simulink model "Torque_Vectoring"  (R2024a)
settings: Solver=FixedStepAuto  StartTime=0.0  StopTime=10.0  FixedStep=0.01  RelTol=1e-3
model workspace (MAT data in the model file):
  diff_table_F = [0 0.0005 0.0005 0.0006 0.0006 0.0007 0.0008 0.0008 0.0009 0.0009 0.001 0.0011 0.0011 0.0012 0.0013 0.0014 0.0014 0.0015 0.0016 0.0017 0.0018 0.0018 0.0019 0.002 0.0021 0.0022 0.0023 0.0024 0.0025 0.0026 0.0027 0.0027 0.0028 0.0029 0.0031 0.0032 0.0033 0.0034 0.0035 0.0036 0.0037 0.0038 0.0039 0.004 0.0042 0.0043 0.0044 0.0045 0.0046 0.0048 0.0049 0.005 0.0051 0.0053 0.0054 0.0055 0.0057 0.0058 0.0059 0.0061 0.0062 0.0064 0.0065 0.0067 0.0068 0.007 0.0071 0.0073 0.0074 0.0076 0.0077 0.0079 0.008 0.0082 0.0084 0.0085 0.0087 0.0089 0.009 0.0092 0.0094 0.0095]
  diff_table_R = [0 0.0023 0.00253 0.00276 0.00299 0.00322 0.00345 0.00368 0.00391 0.00414 0.00437 0.0046 0.00483 0.00506 0.00529 0.00552 0.00575 0.00598 0.00621 0.00644 0.00667 0.0069 0.00713 0.00736 0.00759 0.00782 0.00805 0.00828 0.00851 0.00874 0.00897 0.0092 0.00943 0.00966 0.00989 0.01012 0.01035 0.01058 0.01081 0.01104 0.01127 0.0115 0.01173 0.01196 0.01219 0.01242 0.01265 0.01288 0.01311 0.01334 0.01357 0.0138 0.01403 0.01426 0.01449 0.01472 0.01495 0.01518 0.01541 0.01564 0.01587 0.0161 0.01633 0.01656 0.01679 0.01702 0.01725 0.01748 0.01771 0.01794 0.01817 0.0184 0.01863 0.01886 0.01909 0.01932 0.01955 0.01978 0.02001 0.02024 0.02047 0.0207]
  diff_table_ext_F = [0 0.0005 0.0005 0.0006 0.0006 0.0007 0.0008 0.0008 0.0009 0.0009 0.001 0.0011 0.0011 0.0012 0.0013 0.0014 0.0014 0.0015 0.0016 0.0017 0.0018 0.0018 0.0019 0.002 0.0021 0.0022 0.0023 0.0024 0.0025 0.0026 0.0027 0.0027 0.0028 0.0029 0.0031 0.0032 0.0033 0.0034 0.0035 0.0036 0.0037 0.0038 0.0039 0.004 0.0042 0.0043 0.0044 0.0045 0.0046 0.0048 0.0049 0.005 0.0051 0.0053 0.0054 0.0055 0.0057 0.0058 0.0059 0.0061 0.0062 0.0064 0.0065 0.0067 0.0068 0.007 0.0071 0.0073 0.0074 0.0076 0.0077 0.0079 0.008 0.0082 0.0084 0.0085 0.0087 0.0089 0.009 0.0092 0.0094 0.0095 0.0097 0.0099 0.01 0.0102 0.0104 0.0105 0.0107 0.0109 0.011 0.0112 0.0114 0.0115 0.0117 0.0119 0.012 0.0122 0.0124 0.0125 0.0127]
  diff_table_ext_R = [0 0.0023 0.00253 0.00276 0.00299 0.00322 0.00345 0.00368 0.00391 0.00414 0.00437 0.0046 0.00483 0.00506 0.00529 0.00552 0.00575 0.00598 0.00621 0.00644 0.00667 0.0069 0.00713 0.00736 0.00759 0.00782 0.00805 0.00828 0.00851 0.00874 0.00897 0.0092 0.00943 0.00966 0.00989 0.01012 0.01035 0.01058 0.01081 0.01104 0.01127 0.0115 0.01173 0.01196 0.01219 0.01242 0.01265 0.01288 0.01311 0.01334 0.01357 0.0138 0.01403 0.01426 0.01449 0.01472 0.01495 0.01518 0.01541 0.01564 0.01587 0.0161 0.01633 0.01656 0.01679 0.01702 0.01725 0.01748 0.01771 0.01794 0.01817 0.0184 0.01863 0.01886 0.01909 0.01932 0.01955 0.01978 0.02001 0.02024 0.02047 0.0207 0.02093 0.02116 0.02139 0.02162 0.02185 0.02208 0.02231 0.02254 0.02277 0.023 0.02323 0.02346 0.02369 0.02392 0.02415 0.02438 0.02461 0.02484 0.02507]
undefined symbols (not defined in the file): accX, accY, amk_actual_speed, base_torques, dash_se, diff_gain_n, diff_gain_outer, fl, fr, gyrZ, max_torque_front, max_torque_rear, min_torque_front, min_torque_rear, newsignal1, rl, rr, te_main_APPS, te_main_BPSe, torque_front_n, torque_front_p, torque_rear_n, torque_rear_p, yrc_diff_gain, yrc_grip, yrc_ki, yrc_kp_acc, yrc_kp_regen, yrc_ku, yrc_lambda1, yrc_lambda2, yrc_lambda3, yrc_max_power, yrc_steer_factor
libraries: simulink_extras x1, slpidlib x1
settings Model: Creator=andre  LastModifiedBy=pedro
settings OptimizationCC: ZeroExternalMemoryAtStartup=off  ZeroInternalMemoryAtStartup=off
settings RTWCC: Toolchain=Colcon Tools  TargetLang=C++
settings GRTTargetCC: TargetLangStandard=C++11 (ISO)  CodeInterfacePackaging=C++ class  MultiInstanceErrorCode=Warning

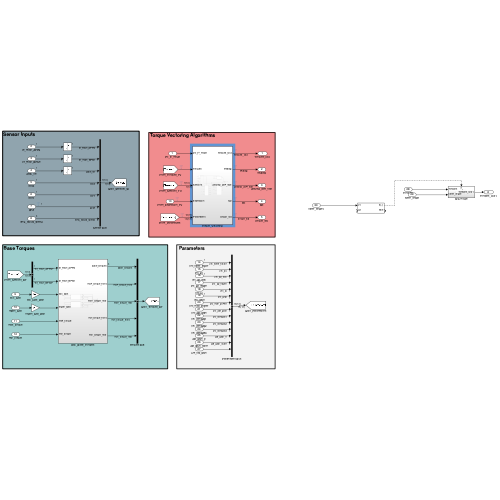
[thumbnail: Simulink's stored preview of the top-level diagram]
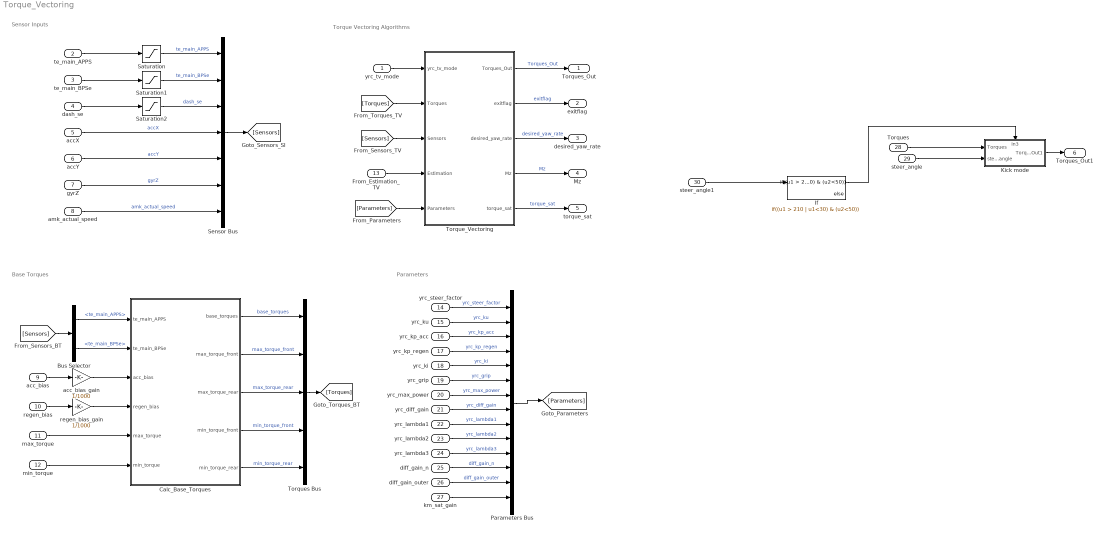
== system Torque_Vectoring ==
  note: Parameters
  note: Base Torques
  note: Torque Vectoring Algorithms
  note: Sensor Inputs
  yrc_tv_mode : Inport
  te_main_APPS : Inport  Port=2  PortDimensions=1
  te_main_BPSe : Inport  Port=3  PortDimensions=1
  dash_se : Inport  Port=4  PortDimensions=1
  accX : Inport  Port=5  PortDimensions=1
  accY : Inport  Port=6  PortDimensions=1
  gyrZ : Inport  Port=7  PortDimensions=1
  amk_actual_speed : Inport  Port=8  PortDimensions=4
  acc_bias : Inport  Port=9
  regen_bias : Inport  Port=10
  max_torque : Inport  Port=11
  min_torque : Inport  Port=12
  From_Estimation_TV : Inport  Port=13
  yrc_steer_factor : Inport  Port=14  PortDimensions=1
  yrc_ku : Inport  Port=15  PortDimensions=1
  yrc_kp_acc : Inport  Port=16  PortDimensions=1
  yrc_kp_regen : Inport  Port=17  PortDimensions=1
  yrc_ki : Inport  Port=18  PortDimensions=1
  yrc_grip : Inport  Port=19  PortDimensions=1
  yrc_max_power : Inport  Port=20  PortDimensions=1
  yrc_diff_gain : Inport  Port=21  PortDimensions=1
  yrc_lambda1 : Inport  Port=22  PortDimensions=1
  yrc_lambda2 : Inport  Port=23  PortDimensions=1
  yrc_lambda3 : Inport  Port=24  PortDimensions=1
  diff_gain_n : Inport  Port=25  PortDimensions=1
  diff_gain_outer : Inport  Port=26  PortDimensions=1
  km_sat_gain : Inport  Port=27
  Torques : Inport  Port=28
  steer_angle : Inport  Port=29
  steer_angle1 : Inport  Port=30
  Bus Selector : BusSelector  OutputSignals=te_main_APPS,te_main_BPSe
  Calc_Base_Torques : Subsystem
  If : If  NumInputs=2  IfExpression=(u1 > 210 | u1<30) & (u2<50)
  Kick mode : Subsystem
      settings: PortSchema="{\"entries\":[{\"content\":{\"sides\":[{\"content\":{\"connectorIds\":[\"In1\",\"In2\"]},\"type\":\"ConnectorPlacement.EquallySpacedRectSide\",\"uuid\":\"e9897e70-c7c7-4947-a7d8-b7fe2c92736f\"},{\"content\":{\"connectorIds\":[\"Out1\"],\"side\":\"RIGHT\"},\"type\":\"ConnectorPlacement.EquallySpacedRectSide\",\"uuid\":\"5825815b-03a9-422c-b961-b03bf00c9827\"},{\"content\":{\"connectorIds\":[\"In3\"],\"side\":\"TOP\"},\"type\":\"ConnectorPlacement.EquallySpacedRectSide\",\"uuid\":\"e2faf393-33b7-422a-8f4d-99abbde724a7\"}]},\"type\":\"ConnectorPlacement.EquallySpacedConnector\",\"uuid\":\"5fc9237a-4862-4d27-81be-376c484d3dd1\"}],\"packageUris\":[\"http://schema.mathworks.com/mf0/Connector/R2020b\"],\"version\":\"1.0\"}"
  Parameters Bus : BusCreator  Inputs=yrc_steer_factor,yrc_ku,yrc_kp_acc,yrc_kp_regen,yrc_ki,yrc_grip,yrc_max_power,yrc_diff_gain,yrc_lambda1,yrc_lambda2,yrc_lambda3,diff_gain_n,diff_gain_outer,newsignal1
  Saturation : Saturate  UpperLimit=100  LowerLimit=0
  Saturation1 : Saturate  UpperLimit=100  LowerLimit=0
  Saturation2 : Saturate  UpperLimit=127  LowerLimit=-127
  Sensor Bus : BusCreator  Inputs=te_main_APPS,te_main_BPSe,dash_se,accX,accY,gyrZ,amk_actual_speed
  Torque_Vectoring : Subsystem
  Torques Bus : BusCreator  Inputs=base_torques,max_torque_front,max_torque_rear,min_torque_front,min_torque_rear
  acc_bias_gain : Gain  Gain=1/1000
  regen_bias_gain : Gain  Gain=1/1000
  Torques_Out : Outport
  exitflag : Outport  Port=2
  desired_yaw_rate : Outport  Port=3
  Mz : Outport  Port=4
  torque_sat : Outport  Port=5
  Torques_Out1 : Outport  Port=6
  wires:
  amk_actual_speed/1 -> Sensor Bus/7  "amk_actual_speed"
  Sensor Bus/1 -> [Sensors]
  yrc_grip/1 -> Parameters Bus/6  "yrc_grip"
  [Parameters] -> Torque_Vectoring/5(Parameters)
  [Torques] -> Torque_Vectoring/2(Torques)
  Torque_Vectoring/3(desired_yaw_rate) -> desired_yaw_rate/1  "desired_yaw_rate"
  regen_bias_gain/1 -> Calc_Base_Torques/4(regen_bias)
  Calc_Base_Torques/5(min_torque_rear) -> Torques Bus/5  "min_torque_rear"
  Calc_Base_Torques/4(min_torque_front) -> Torques Bus/4  "min_torque_front"
  yrc_max_power/1 -> Parameters Bus/7  "yrc_max_power"
  Bus Selector/1 -> Calc_Base_Torques/1(te_main_APPS)  "<te_main_APPS>"
  accY/1 -> Sensor Bus/5  "accY"
  Torque_Vectoring/5(torque_sat) -> torque_sat/1  "torque_sat"
  [Sensors] -> Bus Selector/1
  yrc_kp_regen/1 -> Parameters Bus/4  "yrc_kp_regen"
  Calc_Base_Torques/1(base_torques) -> Torques Bus/1  "base_torques"
  yrc_tv_mode/1 -> Torque_Vectoring/1(yrc_tv_mode)
  [Sensors] -> Torque_Vectoring/3(Sensors)
  Torques Bus/1 -> [Torques]
  regen_bias/1 -> regen_bias_gain/1
  Saturation1/1 -> Sensor Bus/2  "te_main_BPSe"
  dash_se/1 -> Saturation2/1
  yrc_ki/1 -> Parameters Bus/5  "yrc_ki"
  yrc_steer_factor/1 -> Parameters Bus/1  "yrc_steer_factor"
  min_torque/1 -> Calc_Base_Torques/6(min_torque)
  acc_bias/1 -> acc_bias_gain/1
  acc_bias_gain/1 -> Calc_Base_Torques/3(acc_bias)
  Calc_Base_Torques/2(max_torque_front) -> Torques Bus/2  "max_torque_front"
  te_main_APPS/1 -> Saturation/1
  Calc_Base_Torques/3(max_torque_rear) -> Torques Bus/3  "max_torque_rear"
  From_Estimation_TV/1 -> Torque_Vectoring/4(Estimation)
  Saturation/1 -> Sensor Bus/1  "te_main_APPS"
  yrc_kp_acc/1 -> Parameters Bus/3  "yrc_kp_acc"
  gyrZ/1 -> Sensor Bus/6  "gyrZ"
  Parameters Bus/1 -> [Parameters]
  Saturation2/1 -> Sensor Bus/3  "dash_se"
  accX/1 -> Sensor Bus/4  "accX"
  Bus Selector/2 -> Calc_Base_Torques/2(te_main_BPSe)  "<te_main_BPSe>"
  max_torque/1 -> Calc_Base_Torques/5(max_torque)
  te_main_BPSe/1 -> Saturation1/1
  Torque_Vectoring/4(Mz) -> Mz/1  "Mz"
  Torque_Vectoring/2(exitflag) -> exitflag/1  "exitflag"
  yrc_diff_gain/1 -> Parameters Bus/8  "yrc_diff_gain"
  yrc_ku/1 -> Parameters Bus/2  "yrc_ku"
  yrc_lambda1/1 -> Parameters Bus/9  "yrc_lambda1"
  yrc_lambda2/1 -> Parameters Bus/10  "yrc_lambda2"
  yrc_lambda3/1 -> Parameters Bus/11  "yrc_lambda3"
  diff_gain_n/1 -> Parameters Bus/12  "diff_gain_n"
  diff_gain_outer/1 -> Parameters Bus/13  "diff_gain_outer"
  Torque_Vectoring/1(Torques_Out) -> Torques_Out/1  "Torques_Out"
  km_sat_gain/1 -> Parameters Bus/14
  steer_angle1/1 -> If/1
  Kick mode/1(Torques_Out1) -> Torques_Out1/1
  If/1 -> Kick mode/3(In3)
  steer_angle/1 -> Kick mode/2(steer_angle)
  Torques/1 -> Kick mode/1(Torques)

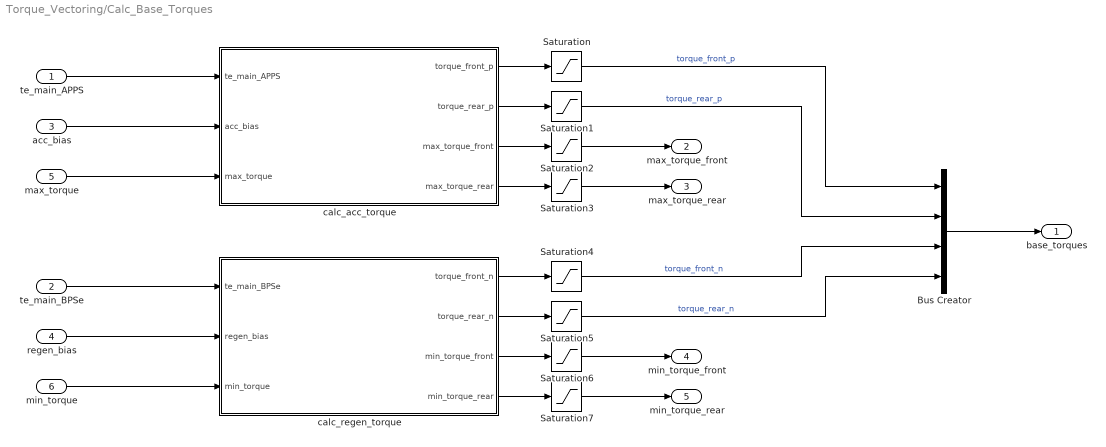
== system Torque_Vectoring/Calc_Base_Torques ==
  te_main_APPS : Inport
  te_main_BPSe : Inport  Port=2
  acc_bias : Inport  Port=3
  regen_bias : Inport  Port=4
  max_torque : Inport  Port=5
  min_torque : Inport  Port=6
  Bus Creator : BusCreator  Inputs=torque_front_p,torque_rear_p,torque_front_n,torque_rear_n
  Saturation{,1..3} (4 alike) : Saturate  UpperLimit=21000  LowerLimit=0
  Saturation{4..7} (4 alike) : Saturate  UpperLimit=0  LowerLimit=-21000
  calc_acc_torque : MATLAB Function  TreatAsAtomicUnit=on
  calc_regen_torque : MATLAB Function  TreatAsAtomicUnit=on
  base_torques : Outport  PortDimensions=4
  max_torque_front : Outport  Port=2
  max_torque_rear : Outport  Port=3
  min_torque_front : Outport  Port=4
  min_torque_rear : Outport  Port=5
  wires:
  te_main_APPS/1 -> calc_acc_torque/1(te_main_APPS)
  acc_bias/1 -> calc_acc_torque/2(acc_bias)
  max_torque/1 -> calc_acc_torque/3(max_torque)
  te_main_BPSe/1 -> calc_regen_torque/1(te_main_BPSe)
  regen_bias/1 -> calc_regen_torque/2(regen_bias)
  min_torque/1 -> calc_regen_torque/3(min_torque)
  calc_acc_torque/1(torque_front_p) -> Saturation/1
  calc_acc_torque/2(torque_rear_p) -> Saturation1/1
  calc_acc_torque/3(max_torque_front) -> Saturation2/1
  calc_acc_torque/4(max_torque_rear) -> Saturation3/1
  calc_regen_torque/1(torque_front_n) -> Saturation4/1
  calc_regen_torque/2(torque_rear_n) -> Saturation5/1
  calc_regen_torque/3(min_torque_front) -> Saturation6/1
  calc_regen_torque/4(min_torque_rear) -> Saturation7/1
  Saturation2/1 -> max_torque_front/1
  Saturation3/1 -> max_torque_rear/1
  Saturation6/1 -> min_torque_front/1
  Saturation7/1 -> min_torque_rear/1
  Bus Creator/1 -> base_torques/1
  Saturation/1 -> Bus Creator/1  "torque_front_p"
  Saturation1/1 -> Bus Creator/2  "torque_rear_p"
  Saturation4/1 -> Bus Creator/3  "torque_front_n"
  Saturation5/1 -> Bus Creator/4  "torque_rear_n"

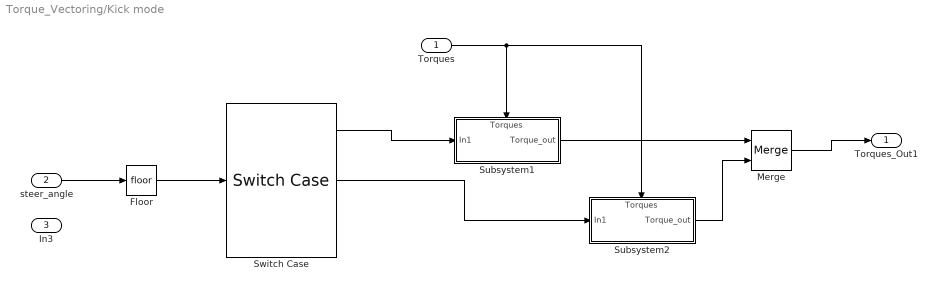
== system Torque_Vectoring/Kick mode ==
  Torques : Inport
  steer_angle : Inport  Port=2
  In3 : Inport  Port=3
  Floor : Rounding
  Merge : Merge
  Subsystem1 : Subsystem
      settings: PortSchema="{\"entries\":[{\"content\":{\"sides\":[{\"content\":{\"connectorIds\":[\"In1\"]},\"type\":\"ConnectorPlacement.EquallySpacedRectSide\",\"uuid\":\"08cef44f-9403-4a7e-80cd-188495bf4ffe\"},{\"content\":{\"connectorIds\":[\"Out1\"],\"side\":\"RIGHT\"},\"type\":\"ConnectorPlacement.EquallySpacedRectSide\",\"uuid\":\"56e69b5d-38a8-4864-8637-0441600913d6\"},{\"content\":{\"connectorIds\":[\"In2\"],\"side\":\"TOP\"},\"type\":\"ConnectorPlacement.EquallySpacedRectSide\",\"uuid\":\"983275be-1625-4fe8-b202-c3acafa806fd\"}]},\"type\":\"ConnectorPlacement.EquallySpacedConnector\",\"uuid\":\"3a10482c-ca03-43ee-b56a-b119a43dac9c\"}],\"packageUris\":[\"http://schema.mathworks.com/mf0/Connector/R2020b\"],\"version\":\"1.0\"}"
  Subsystem2 : Subsystem
      settings: PortSchema="{\"entries\":[{\"content\":{\"sides\":[{\"content\":{\"connectorIds\":[\"In1\"]},\"type\":\"ConnectorPlacement.EquallySpacedRectSide\",\"uuid\":\"08cef44f-9403-4a7e-80cd-188495bf4ffe\"},{\"content\":{\"connectorIds\":[\"Out1\"],\"side\":\"RIGHT\"},\"type\":\"ConnectorPlacement.EquallySpacedRectSide\",\"uuid\":\"56e69b5d-38a8-4864-8637-0441600913d6\"},{\"content\":{\"connectorIds\":[\"In2\"],\"side\":\"TOP\"},\"type\":\"ConnectorPlacement.EquallySpacedRectSide\",\"uuid\":\"983275be-1625-4fe8-b202-c3acafa806fd\"}]},\"type\":\"ConnectorPlacement.EquallySpacedConnector\",\"uuid\":\"3a10482c-ca03-43ee-b56a-b119a43dac9c\"}],\"packageUris\":[\"http://schema.mathworks.com/mf0/Connector/R2020b\"],\"version\":\"1.0\"}"
  Switch Case : SwitchCase  CaseConditions={[210:240],[0:30]}
  Torques_Out1 : Outport
  wires:
  Torques/1 -> Subsystem2/2(Torques), Subsystem1/2(Torques)
  steer_angle/1 -> Floor/1
  Floor/1 -> Switch Case/1
  Switch Case/1 -> Subsystem1/1(In1)
  Switch Case/2 -> Subsystem2/1(In1)
  Subsystem1/1(Torque_out) -> Merge/1
  Subsystem2/1(Torque_out) -> Merge/2
  Merge/1 -> Torques_Out1/1

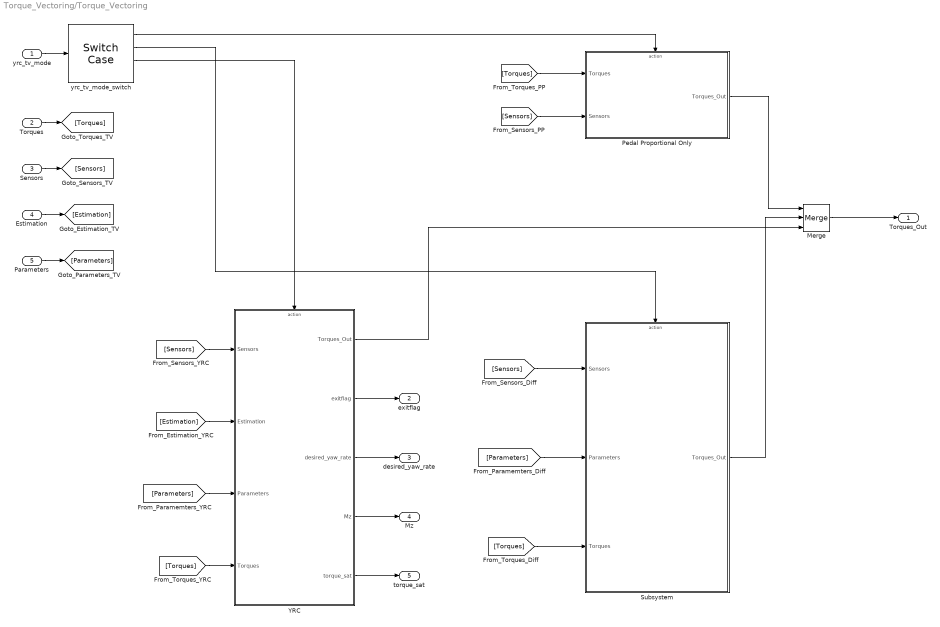
== system Torque_Vectoring/Torque_Vectoring ==
  yrc_tv_mode : Inport
  Torques : Inport  Port=2
  Sensors : Inport  Port=3
  Estimation : Inport  Port=4
  Parameters : Inport  Port=5
  Merge : Merge  Inputs=3
  Pedal Proportional Only : Subsystem
  Subsystem : Subsystem
  YRC : Subsystem
  yrc_tv_mode_switch : SwitchCase  CaseConditions={1,2,3}
  Torques_Out : Outport
  exitflag : Outport  Port=2
  desired_yaw_rate : Outport  Port=3
  Mz : Outport  Port=4
  torque_sat : Outport  Port=5
  wires:
  Torques/1 -> [Torques]
  Sensors/1 -> [Sensors]
  yrc_tv_mode/1 -> yrc_tv_mode_switch/1
  [Torques] -> Pedal Proportional Only/1(Torques)
  yrc_tv_mode_switch/1 -> Pedal Proportional Only/Action
  [Sensors] -> Pedal Proportional Only/2(Sensors)
  [Sensors] -> YRC/1(Sensors)
  Estimation/1 -> [Estimation]
  [Estimation] -> YRC/2(Estimation)
  Parameters/1 -> [Parameters]
  [Parameters] -> YRC/3(Parameters)
  [Torques] -> YRC/4(Torques)
  YRC/2(exitflag) -> exitflag/1
  YRC/3(desired_yaw_rate) -> desired_yaw_rate/1
  YRC/4(Mz) -> Mz/1
  YRC/5(torque_sat) -> torque_sat/1
  Pedal Proportional Only/1(Torques_Out) -> Merge/1
  YRC/1(Torques_Out) -> Merge/3
  Merge/1 -> Torques_Out/1
  yrc_tv_mode_switch/3 -> YRC/Action
  yrc_tv_mode_switch/2 -> Subsystem/Action
  Subsystem/1(Torques_Out) -> Merge/2
  [Sensors] -> Subsystem/1(Sensors)
  [Torques] -> Subsystem/3(Torques)
  [Parameters] -> Subsystem/2(Parameters)

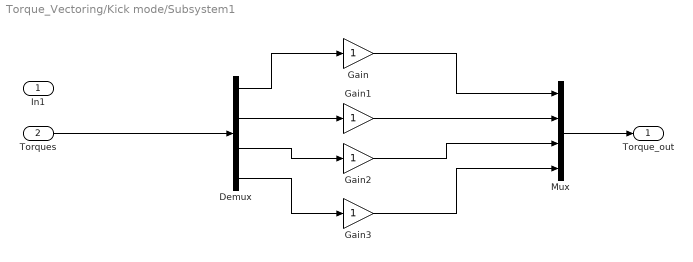
== system Torque_Vectoring/Kick mode/Subsystem1 ==
  In1 : Inport
  Torques : Inport  Port=2
  Demux : Demux
  Gain{,1..3} (4 alike) : Gain
  Mux : Mux
  Torque_out : Outport
  wires:
  Torques/1 -> Demux/1
  Demux/1 -> Gain/1
  Demux/2 -> Gain1/1
  Demux/3 -> Gain2/1
  Demux/4 -> Gain3/1
  Gain/1 -> Mux/1
  Gain1/1 -> Mux/2
  Gain2/1 -> Mux/3
  Gain3/1 -> Mux/4
  Mux/1 -> Torque_out/1

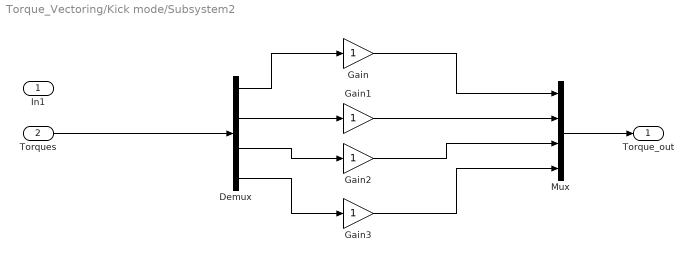
== system Torque_Vectoring/Kick mode/Subsystem2 ==
  In1 : Inport
  Torques : Inport  Port=2
  Demux : Demux
  Gain{,1..3} (4 alike) : Gain
  Mux : Mux
  Torque_out : Outport
  wires:
  Torques/1 -> Demux/1
  Demux/1 -> Gain/1
  Demux/2 -> Gain1/1
  Demux/3 -> Gain2/1
  Demux/4 -> Gain3/1
  Gain/1 -> Mux/1
  Gain1/1 -> Mux/2
  Gain2/1 -> Mux/3
  Gain3/1 -> Mux/4
  Mux/1 -> Torque_out/1

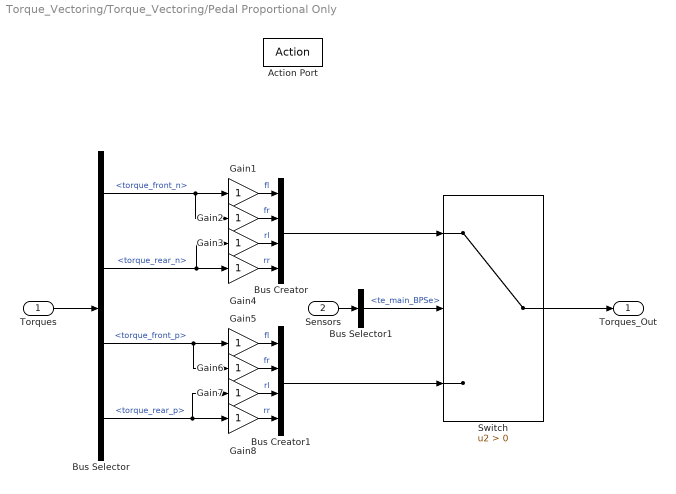
== system Torque_Vectoring/Torque_Vectoring/Pedal Proportional Only ==
  Torques : Inport
  Sensors : Inport  Port=2
  Action Port : ActionPort  ActionPortLabel=case [ 1 ]:
  Bus Creator : BusCreator  Inputs=fl,fr,rl,rr
  Bus Creator1 : BusCreator  Inputs=fl,fr,rl,rr
  Bus Selector : BusSelector  OutputSignals=base_torques.torque_front_n,base_torques.torque_rear_n,base_torques.torque_front_p,base_torques.torque_rear_p
  Bus Selector1 : BusSelector  OutputSignals=te_main_BPSe
  Gain{1..8} (8 alike) : Gain
  Switch : Switch  Criteria=u2 > Threshold  SaturateOnIntegerOverflow=off  InputSameDT=off
  Torques_Out : Outport
  wires:
  Torques/1 -> Bus Selector/1
  Sensors/1 -> Bus Selector1/1
  Switch/1 -> Torques_Out/1
  Bus Selector1/1 -> Switch/2  "<te_main_BPSe>"
  Gain1/1 -> Bus Creator/1  "fl"
  Gain2/1 -> Bus Creator/2  "fr"
  Gain3/1 -> Bus Creator/3  "rl"
  Gain4/1 -> Bus Creator/4  "rr"
  Gain5/1 -> Bus Creator1/1  "fl"
  Gain6/1 -> Bus Creator1/2  "fr"
  Gain7/1 -> Bus Creator1/3  "rl"
  Gain8/1 -> Bus Creator1/4  "rr"
  Bus Selector/1 -> Gain2/1, Gain1/1  "<torque_front_n>"
  Bus Selector/2 -> Gain3/1, Gain4/1  "<torque_rear_n>"
  Bus Selector/3 -> Gain6/1, Gain5/1  "<torque_front_p>"
  Bus Selector/4 -> Gain7/1, Gain8/1  "<torque_rear_p>"
  Bus Creator/1 -> Switch/1
  Bus Creator1/1 -> Switch/3

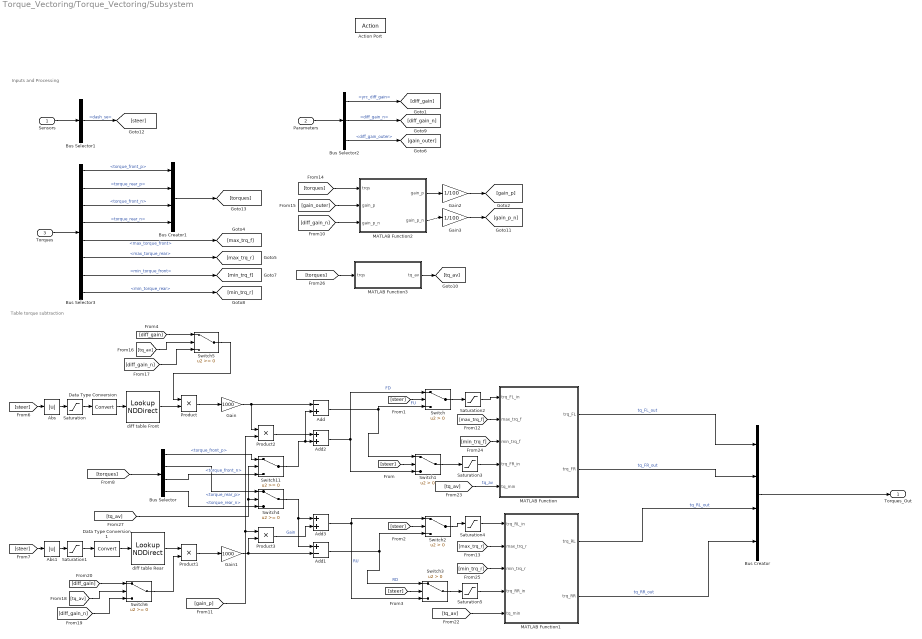
== system Torque_Vectoring/Torque_Vectoring/Subsystem ==
  note: Inputs and Processing
  note: Table torque subtraction
  Sensors : Inport
  Parameters : Inport  Port=2
  Torques : Inport  Port=3
  Action Port : ActionPort  ActionPortLabel=case [ 2 ]:
  Abs : Abs  SaturateOnIntegerOverflow=off
  Abs1 : Abs  SaturateOnIntegerOverflow=off
  Add : Sum  Inputs=-+
  Add1 : Sum  Inputs=+-
  Add2 : Sum
  Add3 : Sum
  Bus Creator : BusCreator  Inputs=4
  Bus Creator1 : BusCreator  Inputs=4
  Bus Selector : BusSelector  OutputSignals=torque_front_p,torque_rear_p,torque_front_n,torque_rear_n
  Bus Selector1 : BusSelector  OutputSignals=dash_se
  Bus Selector2 : BusSelector  OutputSignals=yrc_diff_gain,diff_gain_n,diff_gain_outer
  Bus Selector3 : BusSelector  OutputSignals=base_torques.torque_front_p,base_torques.torque_rear_p,base_torques.torque_front_n,base_torques.torque_rear_n,max_torque_front,max_torque_rear,min_torque_front,min_torque_rear
  Data Type Conversion : DataTypeConversion  SaturateOnIntegerOverflow=off  RndMeth=Floor
  Data Type Conversion1 : DataTypeConversion  SaturateOnIntegerOverflow=off  RndMeth=Floor
  Gain : Gain  Gain=1000
  Gain1 : Gain  Gain=1000
  Gain2 : Gain  Gain=1/100
  Gain3 : Gain  Gain=1/100
  MATLAB Function : MATLAB Function  TreatAsAtomicUnit=on
  MATLAB Function1 : MATLAB Function  TreatAsAtomicUnit=on
  MATLAB Function2 : MATLAB Function  TreatAsAtomicUnit=on
  MATLAB Function3 : MATLAB Function  TreatAsAtomicUnit=on
  Product{,1..3} (4 alike) : Product
  Saturation : Saturate  UpperLimit=100  LowerLimit=0  ZeroCross=off
  Saturation1 : Saturate  UpperLimit=100  LowerLimit=0  ZeroCross=off
  Saturation{2..5} (4 alike) : Saturate  UpperLimit=21000  LowerLimit=-21000  ZeroCross=off
  Switch{,1..3} (4 alike) : Switch  Criteria=u2 > Threshold  SaturateOnIntegerOverflow=off  InputSameDT=off
  Switch{4..6,11} (4 alike) : Switch  SaturateOnIntegerOverflow=off  InputSameDT=off
  diff table Front : LookupNDDirect  NumberOfTableDimensions=1  Table=diff_table_ext_F
  diff table Rear : LookupNDDirect  NumberOfTableDimensions=1  Table=diff_table_ext_R
  Torques_Out : Outport  VectorParamsAs1DForOutWhenUnconnected=off
  wires:
  Bus Selector/4 -> Switch4/3  "<torque_rear_n>"
  [torques] -> Bus Selector/1
  Data Type Conversion/1 -> diff table Front/1
  Saturation3/1 -> MATLAB Function/4(trq_FR_in)
  Add1/1 -> Switch2/3, Switch3/1  "RD"
  Switch11/1 -> Add/2, Add2/2
  [max_trq_r] -> MATLAB Function1/2(max_trq_r)
  Saturation2/1 -> MATLAB Function/1(trq_FL_in)
  Data Type Conversion1/1 -> diff table Rear/1
  Abs1/1 -> Saturation1/1
  Saturation/1 -> Data Type Conversion/1
  Add/1 -> Switch1/1, Switch/3  "FU"
  [steer] -> Switch2/2
  [steer] -> Switch1/2
  [tq_av] -> Switch11/2, Switch4/2
  [gain_outer] -> MATLAB Function2/2("gain_p ")
  [steer] -> Abs/1
  diff table Rear/1 -> Product1/1
  Product/1 -> Gain/1
  MATLAB Function/1(trq_FL) -> Bus Creator/1  "tq_FL_out"
  Switch3/1 -> Saturation5/1
  MATLAB Function2/1(gain_p) -> Gain2/1
  Gain2/1 -> [gain_p]
  Gain/1 -> Add/1, Product2/1
  Bus Selector/1 -> Switch11/1  "<torque_front_p>"
  Switch2/1 -> Saturation4/1
  [gain_p] -> Product2/2, Product3/1
  Switch5/1 -> Product/1
  [min_trq_r] -> MATLAB Function1/3(min_trq_r)
  Switch1/1 -> Saturation3/1
  Saturation1/1 -> Data Type Conversion1/1
  Bus Selector/2 -> Switch4/1  "<torque_rear_p>"
  Saturation5/1 -> MATLAB Function1/4(trq_RR_in)
  Gain1/1 -> Add1/2, Product3/2
  Switch6/1 -> Product1/2
  Abs/1 -> Saturation/1
  [torques] -> MATLAB Function3/1(trqs)
  MATLAB Function3/1(tq_av) -> [tq_av]
  Product1/1 -> Gain1/1
  [steer] -> Switch/2
  Bus Creator/1 -> Torques_Out/1
  diff table Front/1 -> Product/2
  MATLAB Function1/1(trq_RL) -> Bus Creator/3  "tq_RL_out"
  MATLAB Function1/2(trq_RR) -> Bus Creator/4  "tq_RR_out"
  [min_trq_f] -> MATLAB Function/3(min_trq_f)
  [tq_av] -> MATLAB Function/5(tq_min)  "tq_av"
  Saturation4/1 -> MATLAB Function1/1(trq_RL_in)
  [torques] -> MATLAB Function2/1(trqs)
  Add3/1 -> Switch3/3, Switch2/1  "RU"
  [tq_av] -> Switch5/2
  [diff_gain_n] -> Switch6/3
  [steer] -> Switch3/2
  MATLAB Function/2(trq_FR) -> Bus Creator/2  "tq_FR_out"
  [steer] -> Abs1/1
  [max_trq_f] -> MATLAB Function/2(max_trq_f)
  Product2/1 -> Add2/1
  Add2/1 -> Switch1/3, Switch/1  "FD"
  [diff_gain_n] -> Switch5/3
  Bus Selector/3 -> Switch11/3  "<torque_front_n>"
  [diff_gain_n] -> MATLAB Function2/3("gain_p_n ")
  Gain3/1 -> [gain_p_n]
  [tq_av] -> MATLAB Function1/5(tq_min)
  MATLAB Function2/2(gain_p_n) -> Gain3/1
  [diff_gain] -> Switch5/1
  Product3/1 -> Add3/2  "Gain"
  [tq_av] -> Switch6/2
  Switch/1 -> Saturation2/1
  [diff_gain] -> Switch6/1
  Switch4/1 -> Add1/1, Add3/1
  Sensors/1 -> Bus Selector1/1
  Bus Selector1/1 -> [steer]  "<dash_se>"
  Parameters/1 -> Bus Selector2/1
  Bus Selector2/1 -> [diff_gain]  "<yrc_diff_gain>"
  Torques/1 -> Bus Selector3/1
  Bus Selector3/4 -> Bus Creator1/4  "<torque_rear_n>"
  Bus Selector3/3 -> Bus Creator1/3  "<torque_front_n>"
  Bus Selector3/2 -> Bus Creator1/2  "<torque_rear_p>"
  Bus Selector3/1 -> Bus Creator1/1  "<torque_front_p>"
  Bus Creator1/1 -> [torques]
  Bus Selector3/8 -> [min_trq_r]  "<min_torque_rear>"
  Bus Selector3/7 -> [min_trq_f]  "<min_torque_front>"
  Bus Selector3/5 -> [max_trq_f]  "<max_torque_front>"
  Bus Selector3/6 -> [max_trq_r]  "<max_torque_rear>"
  Bus Selector2/3 -> [gain_outer]  "<diff_gain_outer>"
  Bus Selector2/2 -> [diff_gain_n]  "<diff_gain_n>"

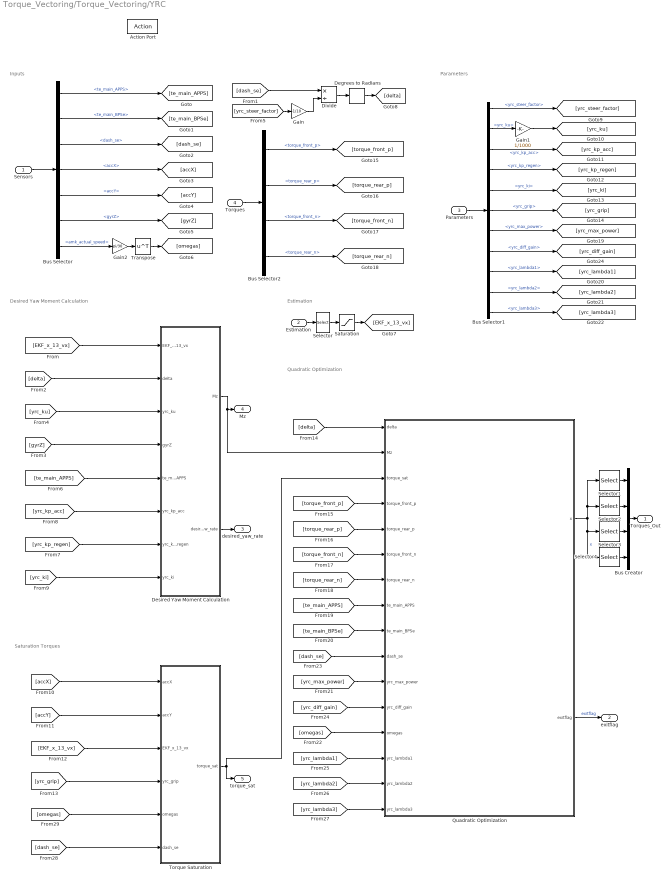
== system Torque_Vectoring/Torque_Vectoring/YRC ==
  note: Inputs
  note: Desired Yaw Moment Calculation
  note: Saturation Torques
  note: Parameters
  note: Estimation
  note: Quadratic Optimization
  Sensors : Inport
  Estimation : Inport  Port=2
  Parameters : Inport  Port=3
  Torques : Inport  Port=4
  Action Port : ActionPort  ActionPortLabel=case [ 3 ]:
  Bus Creator : BusCreator  Inputs=4
  Bus Selector : BusSelector  OutputSignals=te_main_APPS,te_main_BPSe,dash_se,accX,accY,gyrZ,amk_actual_speed
  Bus Selector1 : BusSelector  OutputSignals=yrc_steer_factor,yrc_ku,yrc_kp_acc,yrc_kp_regen,yrc_ki,yrc_grip,yrc_max_power,yrc_diff_gain,yrc_lambda1,yrc_lambda2,yrc_lambda3
  Bus Selector2 : BusSelector  OutputSignals=base_torques.torque_front_p,base_torques.torque_rear_p,base_torques.torque_front_n,base_torques.torque_rear_n
  Degrees to Radians : simulink_extras/Transformations/Degrees to Radians
  Desired Yaw Moment Calculation : Subsystem
  Divide : Product  Inputs=*/
  Gain : Gain  Gain=-1/10
  Gain1 : Gain  Gain=1/1000
  Gain2 : Gain  Gain=pi/30
  Quadratic Optimization : MATLAB Function  TreatAsAtomicUnit=on
  Saturation : Saturate  UpperLimit=35  LowerLimit=0
  Selector : Selector  InputPortWidth=15  IndexOptions=Index vector (dialog)  Indices=[13]  OutputSizes=1
  Selector1 : Selector  InputPortWidth=4  IndexOptions=Index vector (dialog)  Indices=[1]  OutputSizes=1
  Selector2 : Selector  InputPortWidth=4  IndexOptions=Index vector (dialog)  Indices=[2]  OutputSizes=1
  Selector3 : Selector  InputPortWidth=4  IndexOptions=Index vector (dialog)  Indices=[3]  OutputSizes=1
  Selector4 : Selector  InputPortWidth=4  IndexOptions=Index vector (dialog)  Indices=[4]  OutputSizes=1
  Torque Saturation : Subsystem
  Transpose : Math  Operator=transpose
  Torques_Out : Outport
  exitflag : Outport  Port=2
  desired_yaw_rate : Outport  Port=3
  Mz : Outport  Port=4
  torque_sat : Outport  Port=5
  wires:
  Sensors/1 -> Bus Selector/1
  Bus Selector/1 -> [te_main_APPS]  "<te_main_APPS>"
  Bus Selector/2 -> [te_main_BPSe]  "<te_main_BPSe>"
  Bus Selector/3 -> [dash_se]  "<dash_se>"
  Bus Selector/4 -> [accX]  "<accX>"
  Bus Selector/5 -> [accY]  "<accY>"
  Bus Selector/6 -> [gyrZ]  "<gyrZ>"
  Bus Selector/7 -> Gain2/1  "<amk_actual_speed>"
  Estimation/1 -> Selector/1
  Selector/1 -> Saturation/1
  Saturation/1 -> [EKF_x_13_vx]
  [EKF_x_13_vx] -> Desired Yaw Moment Calculation/1(EKF_x_13_vx)
  [dash_se] -> Divide/1
  [delta] -> Desired Yaw Moment Calculation/2(delta)
  Parameters/1 -> Bus Selector1/1
  Bus Selector1/1 -> [yrc_steer_factor]  "<yrc_steer_factor>"
  [yrc_ku] -> Desired Yaw Moment Calculation/3(yrc_ku)
  Bus Selector1/2 -> Gain1/1  "<yrc_ku>"
  Gain1/1 -> [yrc_ku]
  [yrc_steer_factor] -> Gain/1
  Gain/1 -> Divide/2
  Divide/1 -> Degrees to Radians/1
  Degrees to Radians/1 -> [delta]
  [gyrZ] -> Desired Yaw Moment Calculation/4(gyrZ)
  [te_main_APPS] -> Desired Yaw Moment Calculation/5(te_main_APPS)
  Bus Selector1/3 -> [yrc_kp_acc]  "<yrc_kp_acc>"
  Bus Selector1/4 -> [yrc_kp_regen]  "<yrc_kp_regen>"
  [yrc_kp_acc] -> Desired Yaw Moment Calculation/6(yrc_kp_acc)
  [yrc_kp_regen] -> Desired Yaw Moment Calculation/7(yrc_kp_regen)
  Bus Selector1/5 -> [yrc_ki]  "<yrc_ki>"
  [yrc_ki] -> Desired Yaw Moment Calculation/8(yrc_ki)
  [accY] -> Torque Saturation/2(accY)
  [accX] -> Torque Saturation/1(accX)
  [EKF_x_13_vx] -> Torque Saturation/3(EKF_x_13_vx)
  [yrc_grip] -> Torque Saturation/4(yrc_grip)
  Bus Selector1/6 -> [yrc_grip]  "<yrc_grip>"
  [delta] -> Quadratic Optimization/1(delta)
  Desired Yaw Moment Calculation/1(Mz) -> Quadratic Optimization/2(Mz), Mz/1
  Torque Saturation/1(torque_sat) -> Quadratic Optimization/3(torque_sat), torque_sat/1
  Torques/1 -> Bus Selector2/1
  Bus Selector2/1 -> [torque_front_p]  "<torque_front_p>"
  Bus Selector2/4 -> [torque_rear_n]  "<torque_rear_n>"
  Bus Selector2/3 -> [torque_front_n]  "<torque_front_n>"
  Bus Selector2/2 -> [torque_rear_p]  "<torque_rear_p>"
  [torque_front_p] -> Quadratic Optimization/4(torque_front_p)
  [torque_rear_p] -> Quadratic Optimization/5(torque_rear_p)
  [torque_front_n] -> Quadratic Optimization/6(torque_front_n)
  [torque_rear_n] -> Quadratic Optimization/7(torque_rear_n)
  [te_main_APPS] -> Quadratic Optimization/8(te_main_APPS)
  [te_main_BPSe] -> Quadratic Optimization/9(te_main_BPSe)
  Bus Selector1/7 -> [yrc_max_power]  "<yrc_max_power>"
  [yrc_max_power] -> Quadratic Optimization/11(yrc_max_power)
  Transpose/1 -> [omegas]
  Gain2/1 -> Transpose/1
  [omegas] -> Quadratic Optimization/13(omegas)
  [dash_se] -> Quadratic Optimization/10(dash_se)
  Bus Selector1/8 -> [yrc_diff_gain]  "<yrc_diff_gain>"
  [yrc_diff_gain] -> Quadratic Optimization/12(yrc_diff_gain)
  Quadratic Optimization/2(exitflag) -> exitflag/1  "exitflag"
  Quadratic Optimization/1(x) -> Selector1/1, Selector2/1, Selector3/1, Selector4/1  "x"
  Bus Creator/1 -> Torques_Out/1
  Selector1/1 -> Bus Creator/1
  Selector2/1 -> Bus Creator/2
  Selector3/1 -> Bus Creator/3
  Selector4/1 -> Bus Creator/4
  Desired Yaw Moment Calculation/2(desired_yaw_rate) -> desired_yaw_rate/1
  Bus Selector1/9 -> [yrc_lambda1]  "<yrc_lambda1>"
  Bus Selector1/10 -> [yrc_lambda2]  "<yrc_lambda2>"
  Bus Selector1/11 -> [yrc_lambda3]  "<yrc_lambda3>"
  [yrc_lambda1] -> Quadratic Optimization/14(yrc_lambda1)
  [yrc_lambda2] -> Quadratic Optimization/15(yrc_lambda2)
  [yrc_lambda3] -> Quadratic Optimization/16(yrc_lambda3)
  [dash_se] -> Torque Saturation/6(dash_se)
  [omegas] -> Torque Saturation/5(omegas)

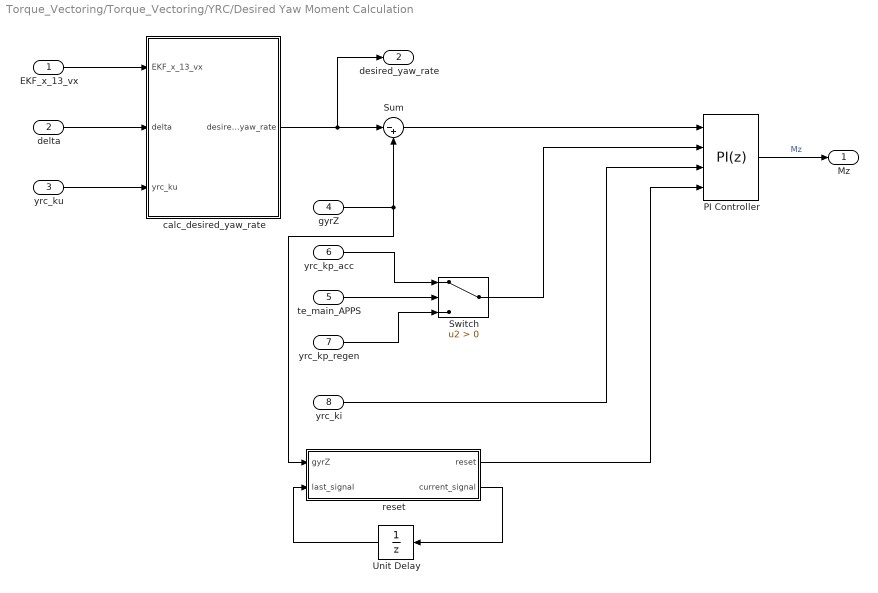
== system Torque_Vectoring/Torque_Vectoring/YRC/Desired Yaw Moment Calculation ==
  EKF_x_13_vx : Inport
  delta : Inport  Port=2
  yrc_ku : Inport  Port=3  PortDimensions=1
  gyrZ : Inport  Port=4  PortDimensions=1
  te_main_APPS : Inport  Port=5  PortDimensions=1
  yrc_kp_acc : Inport  Port=6  PortDimensions=1
  yrc_kp_regen : Inport  Port=7  PortDimensions=1
  yrc_ki : Inport  Port=8  PortDimensions=1
  PI Controller : slpidlib/PID Controller  Controller=PI  Form=Parallel  TimeDomain=Discrete-time  UseExternalTs=off  SampleTime=-1  IntegratorMethod=Backward Euler  FilterMethod=Forward Euler  ControllerParametersSource=external  P=400  I=100  UseKiTs=off  D=10  UseExternalDerivativeSource=off  N=1  UseFilter=on  TunerSelectOption=Transfer Function Based (PID Tuner App)  InitialConditionSource=internal  InitialConditionForIntegrator=0  InitialConditionForFilter=0  DifferentiatorICPrevScaledInput=0  ExternalReset=rising  TrackingMode=off  Kt=1  LimitOutput=on  SatLimitsSource=internal  UpperSaturationLimit=1700  LowerSaturationLimit=-1700  LinearizeAsGain=off  AntiWindupMode=clamping  Kb=6  LimitIntegrator=off  UpperIntegratorSaturationLimit=inf  LowerIntegratorSaturationLimit=-inf  POutMin=[]  POutMax=[]  IOutMin=[]  IOutMax=[]  DOutMin=[]  DOutMax=[]  NOutMin=[]  NOutMax=[]  SumOutMin=[]  SumOutMax=[]  SaturationOutMin=[]  SaturationOutMax=[]  PParamMin=[]  PParamMax=[]  IParamMin=[]  IParamMax=[]  DParamMin=[]  DParamMax=[]  NParamMin=[]  NParamMax=[]  KbParamMin=[]  KbParamMax=[]  KtParamMin=[]  KtParamMax=[]  KbOutMin=[]  KbOutMax=[]  KtOutMin=[]  KtOutMax=[]  IntegratorOutMin=[]  IntegratorOutMax=[]  FilterOutMin=[]  FilterOutMax=[]  SumI1OutMin=[]  SumI1OutMax=[]  SumI2OutMin=[]  SumI2OutMax=[]  SumI3OutMin=[]  SumI3OutMax=[]  SumI4OutMin=[]  SumI4OutMax=[]  SumDOutMin=[]  SumDOutMax=[]  DifferentiatorOutMin=[]  DifferentiatorOutMax=[]  FilterDiffOutCoefMin=[]  FilterDiffOutCoefMax=[]  ReciprocalOutMin=[]  ReciprocalOutMax=[]  SumDenOutMin=[]  SumDenOutMax=[]  SumNumOutMin=[]  SumNumOutMax=[]  DivideOutMin=[]  DivideOutMax=[]  UdiffTsProdOutMin=[]  UdiffTsProdOutMax=[]  NTsProdOutMin=[]  NTsProdOutMax=[]  UintegralTsProdOutMin=[]  UintegralTsProdOutMax=[]  UngainTsProdOutMin=[]  UngainTsProdOutMax=[]  ClampingZeroOutDataTypeStr=Inherit: Inherit via back propagation  ClampingZeroOutMin=[]  ClampingZeroOutMax=[]  FilterDenConstantOutDataTypeStr=Inherit: Inherit via back propagation  FilterDenConstantOutMin=[]  FilterDenConstantOutMax=[]  PCopyOutDataTypeStr=Inherit: Inherit via back propagation  PCopyOutMin=[]  PCopyOutMax=[]  NCopyOutDataTypeStr=Inherit: Inherit via back propagation  NCopyOutMin=[]  NCopyOutMax=[]  IntegratorContinuousStateAttributes=''  IntegratorStateMustResolveToSignalObject=off  IntegratorRTWStateStorageClass=Auto  FilterContinuousStateAttributes=''  FilterStateMustResolveToSignalObject=off  FilterRTWStateStorageClass=Auto  ParallelPVariant=ExternalParameters  IdealPVariant=Disabled  IVariant=ExternalParameters  DVariant=Disabled  IntegratorVariant=Discrete  SatVariant=Enabled  AWVariant=DiscClampingParallel  PCopyVariant=Disabled  TRVariant=Disabled  FdbkBlocksVariant=Feedback  IdealPFdbkVariant=Passthrough  SatFdbkVariant=Passthrough  DerivativeFilterVariant=Disabled  NVariant=Disabled  NCopyVariant=Disabled_SignalSpec  FilterICVariant=Disabled  IntegratorICVariant=InternalICs  ExternalResetVariant=ExternalReset  TRSumVariant=Passthrough  SumFdbkVariant=Enabled  SumVariant=Sum_PI  TsampFilterVariant=InternalTs  TsampNgainVariant=Passthrough  TsampIntegralVariant=Disabled_SignalSpec  ExternalSaturationOutDataTypeStr=Inherit: Same as second input  DerivativeSourceVariant=Disabled
  Sum : Sum  Inputs=|-+  OutDataTypeStr=double
  Switch : Switch  Criteria=u2 > Threshold  SaturateOnIntegerOverflow=off  InputSameDT=off
  Unit Delay : UnitDelay  SampleTime=-1  HasFrameUpgradeWarning=on
  calc_desired_yaw_rate : MATLAB Function  TreatAsAtomicUnit=on
  reset : MATLAB Function  TreatAsAtomicUnit=on
  Mz : Outport  PortDimensions=1
  desired_yaw_rate : Outport  Port=2  PortDimensions=1
  wires:
  EKF_x_13_vx/1 -> calc_desired_yaw_rate/1(EKF_x_13_vx)
  delta/1 -> calc_desired_yaw_rate/2(delta)
  yrc_ku/1 -> calc_desired_yaw_rate/3(yrc_ku)
  calc_desired_yaw_rate/1(desired_yaw_rate) -> desired_yaw_rate/1, Sum/1
  gyrZ/1 -> reset/1(gyrZ), Sum/2
  Sum/1 -> PI Controller/1
  te_main_APPS/1 -> Switch/2
  yrc_kp_acc/1 -> Switch/1
  yrc_kp_regen/1 -> Switch/3
  Switch/1 -> PI Controller/2
  yrc_ki/1 -> PI Controller/3
  reset/2(current_signal) -> Unit Delay/1
  Unit Delay/1 -> reset/2(last_signal)
  reset/1(reset) -> PI Controller/4
  PI Controller/1 -> Mz/1  "Mz"

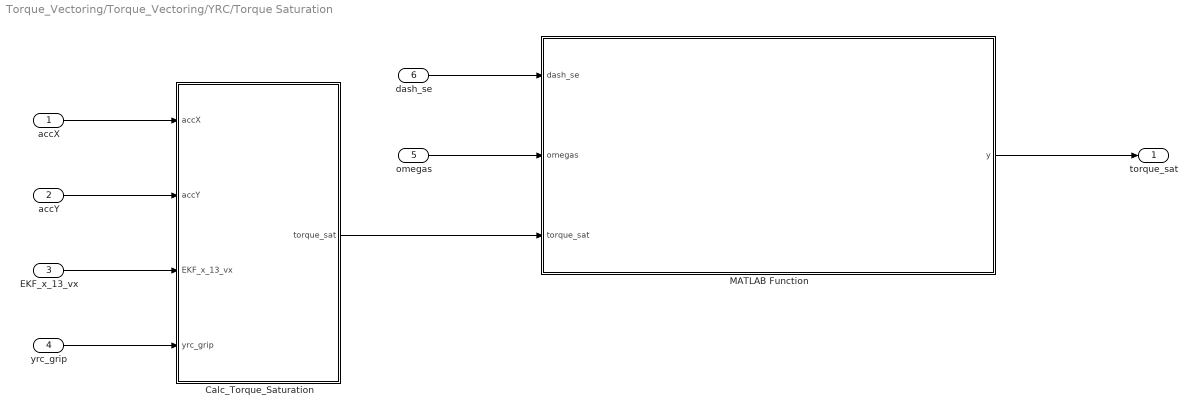
== system Torque_Vectoring/Torque_Vectoring/YRC/Torque Saturation ==
  accX : Inport
  accY : Inport  Port=2
  EKF_x_13_vx : Inport  Port=3
  yrc_grip : Inport  Port=4
  omegas : Inport  Port=5  PortDimensions=4
  dash_se : Inport  Port=6  PortDimensions=1
  Calc_Torque_Saturation : MATLAB Function  TreatAsAtomicUnit=on
  MATLAB Function : MATLAB Function  TreatAsAtomicUnit=on
  torque_sat : Outport  PortDimensions=4
  wires:
  accX/1 -> Calc_Torque_Saturation/1(accX)
  accY/1 -> Calc_Torque_Saturation/2(accY)
  EKF_x_13_vx/1 -> Calc_Torque_Saturation/3(EKF_x_13_vx)
  yrc_grip/1 -> Calc_Torque_Saturation/4(yrc_grip)
  Calc_Torque_Saturation/1(torque_sat) -> MATLAB Function/3(torque_sat)
  MATLAB Function/1(y) -> torque_sat/1
  dash_se/1 -> MATLAB Function/1(dash_se)
  omegas/1 -> MATLAB Function/2(omegas)

== matlab function Torque_Vectoring/Subsystem/MATLAB Function ==
  data: trq_FL_in input; trq_FL output; max_trq_f input; min_trq_f input; trq_FR_in input; trq_FR output; tq_min input
function [trq_FL,trq_FR] = sat(trq_FL_in,max_trq_f,min_trq_f,trq_FR_in,tq_min)
    
    

    if tq_min<0
        trq_FL = max(trq_FL_in,-min_trq_f);
        trq_FR = max(trq_FR_in,-min_trq_f);       
    else
        trq_FL = min(trq_FL_in,max_trq_f);
        trq_FR = min(trq_FR_in,max_trq_f);
    end

    if trq_FL ~= trq_FL_in
       diff=trq_FL_in-trq_FR_in;
       trq_FR=trq_FL-diff;
    elseif trq_FR ~= trq_FR_in
        diff=trq_FR_in - trq_FL_in;
        trq_FL=trq_FR_in -diff;
    end
    
end

== matlab function Torque_Vectoring/YRC/Torque Saturation/MATLAB Function ==
  data: dash_se input; omegas input; torque_sat input; y output
function y = fcn( dash_se ,omegas, torque_sat)

y = u;

== matlab function Torque_Vectoring/Subsystem/MATLAB Function1 ==
  data: trq_RL_in input; trq_RL output; max_trq_r input; min_trq_r input; trq_RR_in input; trq_RR output; tq_min input
function [trq_RL,trq_RR] = sat(trq_RL_in,max_trq_r,min_trq_r,trq_RR_in,tq_min)
    

    if tq_min<0
        trq_RL = max(trq_RL_in,-min_trq_r);
        trq_RR = max(trq_RR_in,-min_trq_r);       
    else
        trq_RL = min(trq_RL_in,max_trq_r);
        trq_RR = min(trq_RR_in,max_trq_r);
    end
    
    if trq_RL ~= trq_RL_in
       diff=trq_RL_in-trq_RR_in;
       trq_RR=trq_RL-diff;
    elseif trq_RR ~= trq_RR_in
        diff=trq_RR_in - trq_RL_in;
        trq_RL=trq_RR_in -diff;
    end
end

== matlab function Torque_Vectoring/Subsystem/MATLAB Function2 ==
  data: trqs input; gain_p output; gain_p input; gain_p_n input; gain_p_n output
function [gain_p,gain_p_n] = fix_tomas(trqs, gain_p,gain_p_n)

% Tomas was dumb and made de walk move forward without APPS
if sum(trqs)==0
    gain_p = 0;
    gain_p_n=0;
end

== matlab function Torque_Vectoring/Subsystem/MATLAB Function3 ==
  data: trqs input; tq_av output
function tq_av= max_torque(trqs)

    trqs=trqs.*1000;
    tq_av=sum(trqs)/4;

== matlab function Torque_Vectoring/Calc_Base_Torques/calc_regen_torque ==
  data: te_main_BPSe input; torque_front_n output double size=1; regen_bias input; min_torque input; torque_rear_n output double size=1; min_torque_front output; min_torque_rear output
function [torque_front_n, torque_rear_n, min_torque_front, min_torque_rear] = ...
    calc_regen_torque(te_main_BPSe, regen_bias, min_torque)

if regen_bias > 0.5
    min_torque_front = - min_torque;
    min_torque_rear = - (min_torque * (1 - regen_bias)) / regen_bias;
else
    min_torque_front = - (min_torque * regen_bias) / (1 - regen_bias);
    min_torque_rear = - min_torque;
end

if te_main_BPSe > 0
    torque_front_n = min_torque_front * (te_main_BPSe / 100);
    torque_rear_n = min_torque_rear * (te_main_BPSe / 100);
else
    torque_front_n = 0;
    torque_rear_n = 0;
end

end

== matlab function Torque_Vectoring/Calc_Base_Torques/calc_acc_torque ==
  data: te_main_APPS input; torque_front_p output size=1; acc_bias input; max_torque input; torque_rear_p output size=1; max_torque_front output; max_torque_rear output
function [torque_front_p, torque_rear_p, max_torque_front, max_torque_rear] = ...
    calc_acc_torque(te_main_APPS, acc_bias, max_torque)

if acc_bias > 0.5
    max_torque_front = max_torque;
    max_torque_rear = (max_torque * (1 - acc_bias)) / acc_bias;
else
    max_torque_front = (max_torque * acc_bias) / (1 - acc_bias);
    max_torque_rear = max_torque;
end

if te_main_APPS > 0
    torque_front_p = max_torque_front * (te_main_mAPPS / 100);
    torque_rear_p = max_torque_rear * (te_main_APPS / 100);
else
    torque_front_p = 0;
    torque_rear_p = 0;
end

end

== matlab function Torque_Vectoring/YRC/Desired Yaw Moment Calculation/calc_desired_yaw_rate ==
  data: EKF_x_13_vx input; desired_yaw_rate output; delta input; yrc_ku input
function desired_yaw_rate = calc_desired_yaw_rate(EKF_x_13_vx, delta, yrc_ku)

wheelbase = 1.54;
desired_yaw_rate = (EKF_x_13_vx * delta) / (wheelbase + yrc_ku*EKF_x_13_vx^2);

== matlab function Torque_Vectoring/YRC/Desired Yaw Moment Calculation/reset ==
  data: gyrZ input; reset output; last_signal input; current_signal output
function [reset, current_signal] = reset(gyrZ, last_signal)

if last_signal == sign(gyrZ)
    reset = 0;
else
    reset = 1;
end
current_signal = sign(gyrZ);
end

== matlab function Torque_Vectoring/YRC/Torque Saturation/Calc_Torque_Saturation ==
  data: accX input; torque_sat output; accY input; EKF_x_13_vx input; yrc_grip input
function torque_sat = calc_torque_saturation(accX, accY, EKF_x_13_vx, yrc_grip)

mass = 302;
wheelbase = 1.54;
track_front = 1.2;
track_rear = 1.2;
height_cg = 0.331;
weight_dist = 0.48;
g = 9.81;
area = 1;
CL = 4.64;
rho = 1.23;
aero_dist = 0.48;
r = 0.235;
GR = 15.21;
mu_x = yrc_grip / 100;
slope_mu = 0.00035;

stationary_front = weight_dist*mass*g;
stationary_rear = (1-weight_dist)*mass*g;

lateral_front = (mass*height_cg*accY)/track_front;
lateral_rear = (mass*height_cg*accY)/track_rear;

longitudinal = (mass*height_cg*accX)/wheelbase;

CL_front = CL*aero_dist;
CL_rear = CL*(1-aero_dist);

lift_front = 0.5*CL_front*rho*EKF_x_13_vx^2*area;
lift_rear = 0.5*CL_rear*rho*EKF_x_13_vx^2*area;

Fz = zeros(4,1);

Fz(1) = stationary_front/2 - longitudinal/2 - lateral_front/2 + lift_front/2;
Fz(2) = stationary_front/2 - longitudinal/2 + lateral_front/2 + lift_front/2;
Fz(3) = stationary_rear/2  + longitudinal/2 - lateral_rear/2  + lift_rear/2;
Fz(4) = stationary_rear/2  + longitudinal/2 + lateral_rear/2  + lift_rear/2;

torque_sat = zeros(4,1);

torque_sat(1) = (Fz(1) * max(mu_x - slope_mu * Fz(1), 1)) / GR * r * 1000;
torque_sat(2) = (Fz(2) * max(mu_x - slope_mu * Fz(2), 1)) / GR * r * 1000;
torque_sat(3) = (Fz(3) * max(mu_x - slope_mu * Fz(3), 1)) / GR * r * 1000;
torque_sat(4) = (Fz(4) * max(mu_x - slope_mu * Fz(4), 1)) / GR * r * 1000;

end

== matlab function Torque_Vectoring/YRC/Quadratic Optimization ==
  data: delta input size=1; Mz input size=1; torque_sat input size=4; torque_front_p input size=1; x output size=[1 4]; exitflag output size=1; torque_rear_p input size=1; torque_front_n input size=1; torque_rear_n input double size=1; te_main_APPS input size=1; te_main_BPSe input size=1; dash_se input size=1; yrc_max_power input size=1; yrc_diff_gain input size=1; omegas input size=4; yrc_lambda1 input size=1; yrc_lambda2 input size=1; yrc_lambda3 input size=1
function [x, exitflag] = quadratic_optimization(delta, Mz, torque_sat,...
    torque_front_p, torque_rear_p, torque_front_n, torque_rear_n,...
    te_main_APPS, te_main_BPSe, dash_se,...
    yrc_max_power, yrc_diff_gain, omegas, yrc_lambda1, yrc_lambda2, yrc_lambda3)

t = 1.2;
wr = 0.235;
a = 0.74;
GR = 15.21;

K = zeros(4,1);
K(1) = (GR / wr) * ((-cos(delta) * t) / 2 + sin(delta) * a);
K(2) = (GR / wr) * (( cos(delta) * t) / 2 + sin(delta) * a);
K(3) = (GR / wr) * (-t / 2);
K(4) = (GR / wr) * ( t / 2);

H1 = K*K';
f = -2*Mz*K;

H2 = diag([1/torque_sat(1)^2, 1/torque_sat(2)^2, 1/torque_sat(3)^2, 1/torque_sat(4)^2]);

H3 = eye(4);

lambda1 = yrc_lambda1;
lambda2 = yrc_lambda2;
lambda3 = yrc_lambda3;

H = lambda1*H1 + lambda2*H2 + lambda3*H3;

if te_main_BPSe == 0

    lb = [0, 0, 0, 0];

    ub = [min(torque_front_p, torque_sat(1)),...
          min(torque_front_p, torque_sat(2)),...
          min(torque_rear_p,  torque_sat(3)),...
          min(torque_rear_p,  torque_sat(4))];

    x0 = ub.*te_main_APPS/100;
    A = [omegas(1),omegas(2),omegas(3),omegas(4)]./1000;
    b = yrc_max_power;

else

    lb = [max(torque_front_n, -torque_sat(1)),...
          max(torque_front_n, -torque_sat(2)),...
          max(torque_rear_n,  -torque_sat(3)),...
          max(torque_rear_n,  -torque_sat(4))];

    ub = [0, 0, 0, 0];
  
    x0 = lb.*te_main_BPSe/100;
    A = -[omegas(1),omegas(2),omegas(3),omegas(4)]./1000;
    b = yrc_max_power;

end

options = optimoptions('quadprog','Algorithm','active-set','Display','off','MaxIterations',500);

[x, ~, exitflag] = quadprog(H, f, A, b, [], [], lb, ub, x0, options);

if exitflag ~= 1
    [x] = differential(lb, ub, te_main_APPS, te_main_BPSe, dash_se, yrc_diff_gain);
end

if te_main_APPS == 0 && te_main_BPSe == 0
    x = x.*0;
end

if te_main_BPSe > 0
    x = min(0, x);
end

end

function [trq] = differential(lb, ub, te_main_APPS, te_main_BPSe, dash_se, yrc_diff_gain)  
    gain = yrc_diff_gain/4;
    if te_main_BPSe == 0
        trq = max(0, ub.*te_main_APPS/100);
        factor = abs(dash_se);
        if dash_se > 0 % turning right
            trq(2)=trq(2)-(trq(2)*(gain/100)*(factor/100));
            trq(4)=trq(4)-(trq(4)*(gain/100)*(factor/100));
        elseif dash_se < 0 % turning left 
            trq(1)=trq(1)-(trq(1)*(gain/100)*(factor/100));
            trq(3)=trq(3)-(trq(3)*(gain/100)*(factor/100));
        end
        trq = max(0,trq); % no negative torques
    else
        trq = min(0, -1.*lb.*te_main_APPS/100); % proportional braking
    end
end
